simulink model "mfunct"  (R2015a)
settings: Solver=ode4  StartTime=0.0  StopTime=15  FixedStep=1e-3  RelTol=1e-3
values from neighbouring files (symbols this model uses):
  b = [1 2 0]'    [Espacio_d_Estados.m]
  k = place(n1,b1,pc)    [dinam19.m]    (also in dinam20.m = place(A,B,pc))
  m = .5    (= 0.5)    [dinam20.m]    (also in dinam21.m; dinam22.m; vparachute.m)
settings Model: Creator=HP  LastModifiedBy=HP

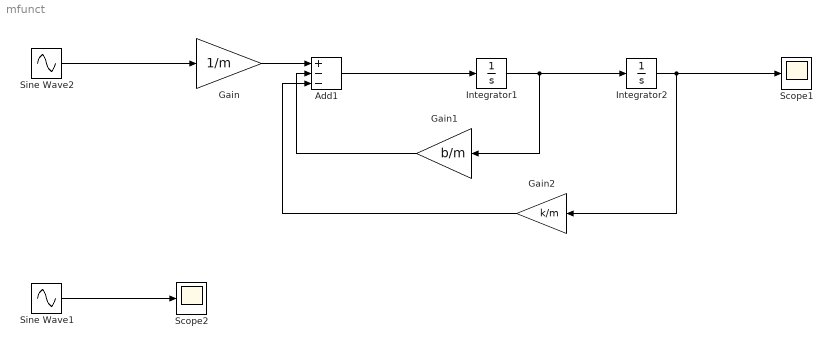
== system mfunct ==
  Add1 : Sum  Inputs=+--
  Gain : Gain  Gain=1/m
  Gain1 : Gain  Gain=b/m
  Gain2 : Gain  Gain=k/m
  Integrator1 : Integrator
  Integrator2 : Integrator
  Scope1 : Scope
  Scope2 : Scope
      settings: YMin=-2  YMax=2
  Sine Wave1 : Sin  Phase=pi/2  SampleTime=0
  Sine Wave2 : Sin  Frequency=2  Phase=pi/2  SampleTime=0
  wires:
  Integrator1/1 -> Gain1/1, Integrator2/1
  Integrator2/1 -> Scope1/1, Gain2/1
  Gain/1 -> Add1/1
  Add1/1 -> Integrator1/1
  Gain1/1 -> Add1/2
  Gain2/1 -> Add1/3
  Sine Wave2/1 -> Gain/1
  Sine Wave1/1 -> Scope2/1
